simulink model "passa_baixa"  (R2024a)
settings: Solver=VariableStepAuto  StartTime=0.0  StopTime=10  RelTol=1e-3
values from neighbouring files (symbols this model uses):
  s = serialport(portaSerial, taxaBits)    [Leitura_analogica_sensor.m]    (also in Leitura_sensor_filtered.m)
libraries: slctrl_linear x1
settings Model: Creator=felliph  LastModifiedBy=felliph
settings DataIOCC: Refine=10

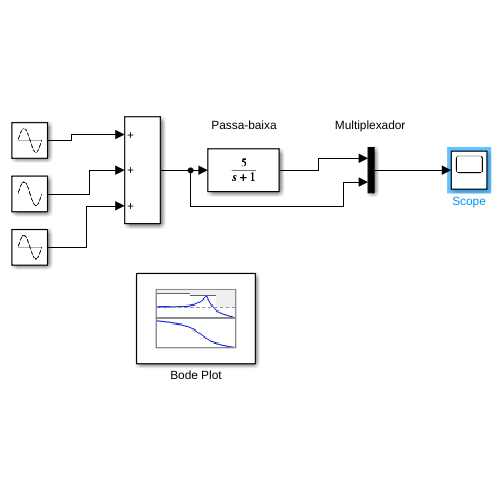
[thumbnail: Simulink's stored preview of the top-level diagram]
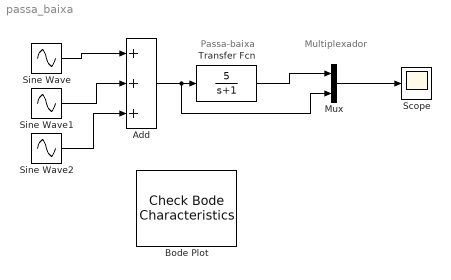
== system passa_baixa ==
  note: Multiplexador
  note: Passa-baixa
  Add : Sum  Inputs=+++
  Bode Plot : slctrl_linear/Check Bode  Characteristics  InstantiateOnLoad=on  SaveOperatingPoints=off  LinearizationIOs={}  LinearizeAt=SnapshotTimes  SnapshotTimes=[0]  TriggerType=rising  SampleTime=auto  RateConversionMethod=zoh  PreWarpFreq=10  UseExactDelayModel=off  UseFullBlockNameLabels=off  UseBusSignalLabels=off  enabled=on  stopWhenAssertionFail=off  export=off  ViewDlgPos=[]  OpenViewOnLoad=off  LaunchViewOnOpen=off  FrequencyUnits=rad/s  MagnitudeUnits=dB  PhaseUnits=deg  TimeUnits=seconds  EnableUpperBound=off  UpperBoundFrequencies=[]  UpperBoundMagnitudes=[]  EnableLowerBound=off  LowerBoundFrequencies=[]  LowerBoundMagnitudes=[]
      settings: LibrarySourceBlock=slctrlblks/Linear Analysis Plots/Bode Plot  SaveToWorkspace=off  SaveName=sys
  Mux : Mux  Inputs=2
  Scope : Scope
  Sine Wave : Sin  Frequency=2*pi*3  SampleTime=0
  Sine Wave1 : Sin  Frequency=2*pi*10  SampleTime=0
  Sine Wave2 : Sin  Frequency=2*pi*50  SampleTime=0
  Transfer Fcn : TransferFcn  Numerator=[5]  Denominator=[1 1]
  wires:
  Mux/1 -> Scope/1
  Transfer Fcn/1 -> Mux/1
  Sine Wave/1 -> Add/1
  Sine Wave1/1 -> Add/2
  Add/1 -> Mux/2, Transfer Fcn/1
  Sine Wave2/1 -> Add/3
